simulink model "TrainSimulation"  (R2020a)
settings: Solver=VariableStepAuto  StartTime=0.0  StopTime=10.0  RelTol=1e-3
values from neighbouring files (symbols this model uses):
  F = 1    [trainparameters.m]
  g = 9.8    [trainparameters.m]
  k = 1    [trainparameters.m]
  M1 = 1    [trainparameters.m]
  M2 = 0.5    [trainparameters.m]
  Mu = 0.02    [trainparameters.m]
settings Model: Creator=diogo  LastModifiedBy=diogo

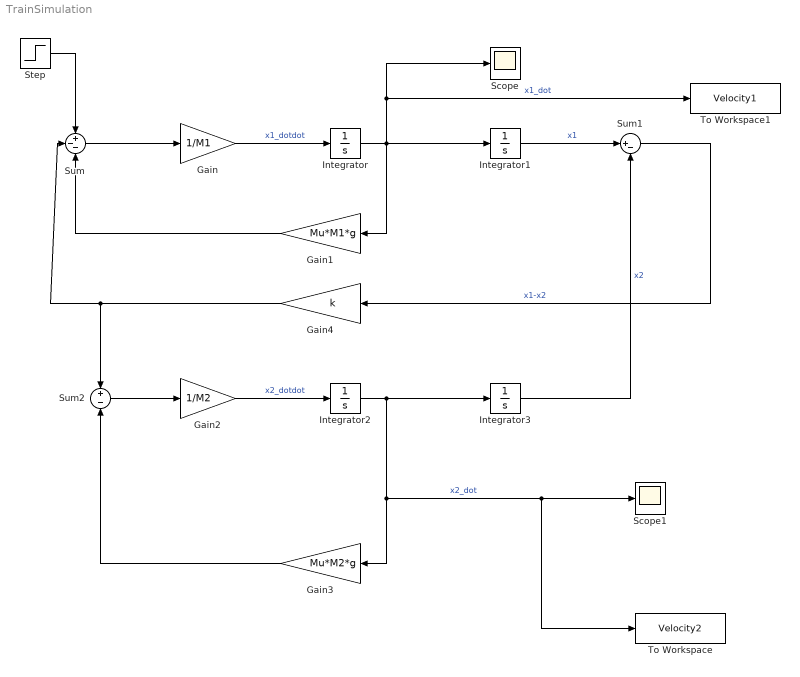
== system TrainSimulation ==
  Gain : Gain  Gain=1/M1
  Gain1 : Gain  Gain=Mu*M1*g
  Gain2 : Gain  Gain=1/M2
  Gain3 : Gain  Gain=Mu*M2*g
  Gain4 : Gain  Gain=k
  Integrator{,1..3} (4 alike) : Integrator
  Scope : Scope
  Scope1 : Scope
  Step : Step  After=F  SampleTime=0
  Sum : Sum  Inputs=+--
  Sum1 : Sum  Inputs=|+-
  Sum2 : Sum  Inputs=+-
  To Workspace : ToWorkspace  VariableName=Velocity2  SaveFormat=Timeseries  SampleTime=-1
  To Workspace1 : ToWorkspace  VariableName=Velocity1  SaveFormat=Timeseries  SampleTime=-1
  wires:
  Gain/1 -> Integrator/1  "x1_dotdot"
  Integrator/1 -> Scope/1, To Workspace1/1, Gain1/1, Integrator1/1  "x1_dot"
  Integrator1/1 -> Sum1/1  "x1"
  Integrator3/1 -> Sum1/2  "x2"
  Integrator2/1 -> Integrator3/1, Gain3/1, To Workspace/1, Scope1/1  "x2_dot"
  Gain2/1 -> Integrator2/1  "x2_dotdot"
  Sum1/1 -> Gain4/1  "x1-x2"
  Step/1 -> Sum/1
  Gain1/1 -> Sum/3
  Gain4/1 -> Sum2/1, Sum/2
  Sum2/1 -> Gain2/1
  Gain3/1 -> Sum2/2
  Sum/1 -> Gain/1
